simulink model "Multiuav"  (Simulink 4.00)
settings: Solver=FixedStepDiscrete  StartTime=0.0  StopTime=g_StopTime  FixedStep=g_SampleTime  RelTol=1e-3
undefined symbols (not defined in the file): ATRFunctions, g_AssignmentAlgorithm, g_CommandTurnRadius, g_CoordinationDelayDen, g_DefaultWaypointAltitude, g_EnableTarget, g_EnableVehicle, g_EntityTypes, g_MaxNumberTargets, g_MaxNumberVehicles, g_MaxReassignmentDeltaTime, g_ObjectMessageIDs, g_OptionSaveDataAVDS, g_OptionSaveDataPlot, g_SampleTime, g_SensorRollLimitDeg, g_TargetStates, g_Tasks, g_TypeAssignment, g_VehicleInputFiles, g_VehicleMemory, g_VehicleTypes, g_WaypointDefinitions, g_WaypointTypes
libraries: cooperative x42
(part 4 of 4)

== system Multiuav/Vehicles/UAV1/EmbeddedFlightSoftware/CooperationManager/Calculate Assignment/CapTransShip/Assignment for Local Vehicle ==
  note: Assignment for Local Vehicle
      |
      | PURPOSE: Output the target and task assignment
      |      for the local vehicle..
      |
      | IMPLEMENTATION: This block uses a"Selector" Block to select the target and task assignment
      |       based on the VehicleID signal.
  note: Note: new assignment is implemented in the route manager.
  In1 : Inport  Port=1  LatchInput=off  SampleTime=g_SampleTime
  In2 : Inport  Port=2  LatchInput=off  SampleTime=g_SampleTime
  Bus Creator : BusCreator  Inputs=3
  Bus Selector : BusSelector  OutputSignals=VehicleID  MuxedOutput=off
  Constant : Constant  Value=0
  Demux : Demux  Outputs=2  BusSelectionMode=off
  SelectedSignals : MATLABFcn  MATLABFcn=[u(1),g_MaxNumberVehicles+u(1)]  OutputDimensions=-1  OutputSignalType=auto  Output1D=on
  Selector : Selector  InputType=Vector  ElementSrc=External  Elements=[1 3]  RowSrc=Internal  Rows=1  ColumnSrc=Internal  Columns=1  InputPortWidth=2*g_MaxNumberVehicles + 1
  Out1 : Outport  Port=1
  wires:
  In1/1 -> Bus Selector/1
  Bus Creator/1 -> Out1/1  "Assignment - Local"
  Demux/1 -> Bus Creator/1  "Target Assignment - Local"
  Demux/2 -> Bus Creator/2  "Task Assignment  - Local"
  Bus Selector/1 -> SelectedSignals/1  "<VehicleID>"
  In2/1 -> Selector/1
  Constant/1 -> Bus Creator/3  "NewAssignmentFlag"
  SelectedSignals/1 -> Selector/2
  Selector/1 -> Demux/1

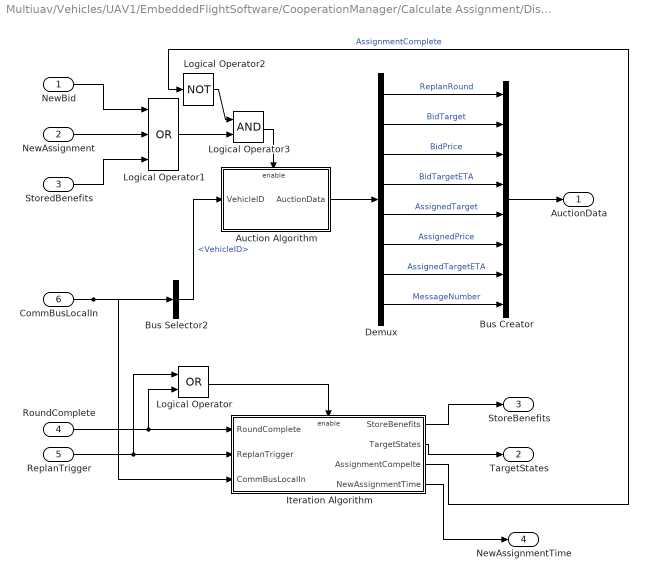
== system Multiuav/Vehicles/UAV1/EmbeddedFlightSoftware/CooperationManager/Calculate Assignment/DistAuctItCapTransShip/Assignment Algorithm ==
  NewBid : Inport  Port=1  LatchInput=off
  NewAssignment : Inport  Port=2  LatchInput=off
  StoredBenefits : Inport  Port=3  LatchInput=off
  RoundComplete : Inport  Port=4  LatchInput=off
  ReplanTrigger : Inport  Port=5  LatchInput=off
  CommBusLocalIn : Inport  Port=6  LatchInput=off
  Auction Algorithm : Subsystem  TreatAsAtomicUnit=on
      settings: RTWFcnNameOpts=Auto  RTWFileNameOpts=Auto
  Bus Creator : BusCreator  Inputs=8
  Bus Selector2 : BusSelector  OutputSignals=VehicleID  MuxedOutput=off
  Demux : Demux  Outputs=[2, g_MaxNumberVehicles,g_MaxNumberVehicles,g_MaxNumberVehicles,g_MaxNumberVehicles,g_MaxNumberVehicles,g_MaxNumberVehicles,1]  BusSelectionMode=off
  Iteration Algorithm : Subsystem  TreatAsAtomicUnit=on
      settings: RTWFcnNameOpts=Auto  RTWFileNameOpts=Auto
  Logical Operator : Logic  Operator=OR  Inputs=2
  Logical Operator1 : Logic  Operator=OR  Inputs=3
  Logical Operator2 : Logic  Operator=NOT  Inputs=21
  Logical Operator3 : Logic  Operator=AND  Inputs=2
  AuctionData : Outport  Port=1
  TargetStates : Outport  Port=2
  StoreBenefits : Outport  Port=3
  NewAssignmentTime : Outport  Port=4
  wires:
  Logical Operator3/1 -> Auction Algorithm/Enable
  Logical Operator2/1 -> Logical Operator3/1
  Logical Operator1/1 -> Logical Operator3/2
  Iteration Algorithm/3(AssignmentCompelte) -> Logical Operator2/1  "AssignmentComplete"
  StoredBenefits/1 -> Logical Operator1/3
  Demux/3 -> Bus Creator/3  "BidPrice"
  Bus Selector2/1 -> Auction Algorithm/1(VehicleID)  "<VehicleID>"
  CommBusLocalIn/1 -> Iteration Algorithm/3(CommBusLocalIn), Bus Selector2/1
  NewBid/1 -> Logical Operator1/1
  NewAssignment/1 -> Logical Operator1/2
  Auction Algorithm/1(AuctionData) -> Demux/1
  Demux/6 -> Bus Creator/6  "AssignedPrice"
  Logical Operator/1 -> Iteration Algorithm/Enable
  RoundComplete/1 -> Logical Operator/2, Iteration Algorithm/1(RoundComplete)
  ReplanTrigger/1 -> Logical Operator/1, Iteration Algorithm/2(ReplanTrigger)
  Iteration Algorithm/2(TargetStates) -> TargetStates/1
  Iteration Algorithm/1(StoreBenefits) -> StoreBenefits/1
  Bus Creator/1 -> AuctionData/1
  Demux/8 -> Bus Creator/8  "MessageNumber"
  Demux/5 -> Bus Creator/5  "AssignedTarget"
  Demux/4 -> Bus Creator/4  "BidTargetETA"
  Demux/2 -> Bus Creator/2  "BidTarget"
  Demux/1 -> Bus Creator/1  "ReplanRound"
  Demux/7 -> Bus Creator/7  "AssignedTargetETA"
  Iteration Algorithm/4(NewAssignmentTime) -> NewAssignmentTime/1

== system Multiuav/Vehicles/UAV1/EmbeddedFlightSoftware/CooperationManager/Calculate Assignment/DistAuctItCapTransShip/Message Processing ==
  CommBusIn : Inport  Port=1  LatchInput=off
  SimBusIn : Inport  Port=2  LatchInput=off
  CommBusLocalIn : Inport  Port=3  LatchInput=off
  ReplanTrigger : Inport  Port=4  LatchInput=off
  Bus Selector1 : BusSelector  OutputSignals=AuctionData  MuxedOutput=off
  Bus Selector2 : BusSelector  OutputSignals=VehicleID  MuxedOutput=off
  Bus Selector4 : BusSelector  OutputSignals=ExternalTruth.VehicleIsDead  MuxedOutput=on
  Demux : Demux  Outputs=[1 1 1]  BusSelectionMode=off
  Logical Operator : Logic  Operator=NOT  Inputs=2
  Mux1 : Mux  Inputs=4
  S-Function : S-Function  FunctionName=DAINF_MessageControlS  PortCounts=[]  SFunctionModules=''
  NewBid : Outport  Port=1
  NewAssignment : Outport  Port=2
  RoundComplete : Outport  Port=3
  wires:
  Demux/3 -> RoundComplete/1
  Demux/2 -> NewAssignment/1
  Demux/1 -> NewBid/1
  S-Function/1 -> Demux/1
  Mux1/1 -> S-Function/1
  Bus Selector2/1 -> Mux1/1  "<VehicleID>"
  CommBusLocalIn/1 -> Bus Selector2/1
  Logical Operator/1 -> Mux1/2  "ActiveVehicles"
  ReplanTrigger/1 -> Mux1/4  "ReplanTrigger"
  Bus Selector1/1 -> Mux1/3  "<AuctionData>"
  CommBusIn/1 -> Bus Selector1/1
  Bus Selector4/1 -> Logical Operator/1  "<VehicleIsDead>"
  SimBusIn/1 -> Bus Selector4/1

== system Multiuav/Vehicles/UAV1/EmbeddedFlightSoftware/CooperationManager/Calculate Assignment/DistAuctItCapTransShip/Replan Logic ==
  EnableType : Inport  Port=1  LatchInput=off
  Constant : Constant  Value=1
  Constant1 : Constant  Value=1
  Constant2 : Constant  Value=0
  Multiport Switch : MultiPortSwitch  Inputs=4
  Sum : Sum  Inputs=++|  SaturateOnIntegerOverflow=on
  ReplanTrigger : Outport  Port=1
  wires:
  Constant1/1 -> Multiport Switch/5, Multiport Switch/3
  Constant2/1 -> Multiport Switch/4, Multiport Switch/2
  Multiport Switch/1 -> ReplanTrigger/1
  Sum/1 -> Multiport Switch/1
  Constant/1 -> Sum/1
  EnableType/1 -> Sum/2

== system Multiuav/Vehicles/UAV1/EmbeddedFlightSoftware/CooperationManager/Calculate Assignment/DistAuctItCapTransShip/Store Benefits ==
  CommBusIn : Inport  Port=1  LatchInput=off
  CommBusLocalIn : Inport  Port=2  LatchInput=off
  TargetStates : Inport  Port=3  LatchInput=off
  Enable : EnablePort  ShowOutputPort=on
  Demux : Demux  Outputs=[g_MaxNumberTargets,g_MaxNumberTargets,1]  BusSelectionMode=off
  Mux : Mux  Inputs=5
  Mux1 : Mux  Inputs=10
  S-Function : S-Function  FunctionName=DINF_CalculateBenefitsS  Parameters=g_MaxNumberTargets,g_MaxNumberVehicles  PortCounts=[]  SFunctionModules=''
  S-Function1 : S-Function  Orientation=left  FunctionName=DAINF_StoreBenefitsS  PortCounts=[]  SFunctionModules=''
  SimBusSelector : BusSelector  OutputSignals=Time,VehicleID,Dynamics(com).AC Dynamics.Position_x,Dynamics(com).AC Dynamics.Position_y,Dynamics(com).AC Dynamics.Psi,Dynamics(com).TacticalManuevering.WayPointNumber,EFS(com).TargetManager(com).SensedTargetInformation.Targets,EFS(com).SensorManager(com).ATR Combined.Desired Headings  MuxedOutput=off
  SimBusSelector1 : BusSelector  OutputSignals=VehicleID  MuxedOutput=off
  SimBusSelector2 : BusSelector  OutputSignals=TriggerReplan  MuxedOutput=off
  BenefitsStored : Outport  Port=1  OutputWhenDisabled=reset  InitialOutput=[0]
  wires:
  SimBusSelector2/1 -> Mux1/10  "<TriggerReplan>"
  CommBusIn/1 -> SimBusSelector2/1
  Enable/1 -> BenefitsStored/1
  SimBusSelector1/1 -> Mux/1  "<VehicleID>"
  Mux/1 -> S-Function1/1
  TargetStates/1 -> Mux/5, Mux1/9  "TargetStates"
  SimBusSelector/6 -> Mux1/6  "<WayPointNumber>"
  SimBusSelector/8 -> Mux1/8  "<Desired Headings>"
  SimBusSelector/7 -> Mux1/7  "<Targets>"
  SimBusSelector/5 -> Mux1/5  "<Psi>"
  SimBusSelector/4 -> Mux1/4  "<Position_y>"
  SimBusSelector/3 -> Mux1/3  "<Position_x>"
  SimBusSelector/2 -> Mux1/2  "<VehicleID>"
  SimBusSelector/1 -> Mux1/1  "<Time>"
  CommBusLocalIn/1 -> SimBusSelector1/1, SimBusSelector/1
  Mux1/1 -> S-Function/1
  S-Function/1 -> Demux/1
  Demux/3 -> Mux/4  "SearchBenefit"
  Demux/2 -> Mux/3  "TimeToComplete"
  Demux/1 -> Mux/2  "TaskBenefits"

== system Multiuav/Vehicles/UAV1/EmbeddedFlightSoftware/CooperationManager/Calculate Assignment/DistItCapTransShip/Assignment Algorithm ==
  ActiveVehicles : Inport  Port=1  LatchInput=off
  ReplanRoundIn : Inport  Port=2  LatchInput=off
  TargetStatesIn : Inport  Port=3  LatchInput=off
  TaskBenefits : Inport  Port=4  LatchInput=off
  TimeToComplete : Inport  Port=5  LatchInput=off
  SearchBenefits : Inport  Port=6  LatchInput=off
  Sync : Inport  Port=7  LatchInput=off
  ReplanTrigger : Inport  Port=8  LatchInput=off
  CommBusLocalIn : Inport  Port=9  LatchInput=off
  Bus Selector : BusSelector  OutputSignals=VehicleID,EFS(com).TargetManager(com).Target Status.TargetStatus,Dynamics(com).TacticalManuevering.WayPointNumber,Dynamics(com).AC Dynamics.Position_x,Dynamics(com).AC Dynamics.Position_y,Dynamics(com).AC Dynamics.Psi  MuxedOutput=off
  Demux : Demux  Outputs=[2 g_MaxNumberTargets 1 1]  BusSelectionMode=off
  Mux : Mux  Inputs=14
  S-Function : S-Function  FunctionName=DINF_CapTransShipAssignS  Parameters=g_MaxNumberTargets,g_MaxNumberVehicles  PortCounts=[]  SFunctionModules=''
  TargetStatesOut : Outport  Port=1
  ReplanRoundOut : Outport  Port=2
  SendBenefitsTrigger : Outport  Port=3
  NewAssignmentTime : Outport  Port=4
  wires:
  Demux/3 -> SendBenefitsTrigger/1
  Bus Selector/6 -> Mux/14  "<Psi>"
  Bus Selector/5 -> Mux/13  "<Position_y>"
  Bus Selector/4 -> Mux/12  "<Position_x>"
  Bus Selector/3 -> Mux/11  "<WayPointNumber>"
  Bus Selector/2 -> Mux/10  "<TargetStatus>"
  Bus Selector/1 -> Mux/9  "<VehicleID>"
  CommBusLocalIn/1 -> Bus Selector/1
  Demux/1 -> ReplanRoundOut/1
  Demux/2 -> TargetStatesOut/1
  S-Function/1 -> Demux/1
  Mux/1 -> S-Function/1
  ReplanTrigger/1 -> Mux/8
  Sync/1 -> Mux/7
  SearchBenefits/1 -> Mux/6
  TimeToComplete/1 -> Mux/5
  TaskBenefits/1 -> Mux/4
  TargetStatesIn/1 -> Mux/3
  ReplanRoundIn/1 -> Mux/2
  ActiveVehicles/1 -> Mux/1
  Demux/4 -> NewAssignmentTime/1

== system Multiuav/Vehicles/UAV1/EmbeddedFlightSoftware/CooperationManager/Calculate Assignment/DistItCapTransShip/Iteration Logic ==
  CommBusIn : Inport  Port=1  LatchInput=off
  SimBusIn : Inport  Port=2  LatchInput=off
  Bus Selector : BusSelector  OutputSignals=ExternalTruth.VehicleIsDead  MuxedOutput=on
  Bus Selector1 : BusSelector  OutputSignals=TaskBenefits  MuxedOutput=off
  Demux : Demux  Outputs=[2,g_MaxNumberTargets,g_MaxNumberVehicles*g_MaxNumberTargets,g_MaxNumberVehicles*g_MaxNumberTargets,g_MaxNumberVehicles,1]  BusSelectionMode=off
  Logical Operator : Logic  Operator=NOT  Inputs=2
  Mux1 : Mux  Inputs=2
  S-Function : S-Function  FunctionName=DINF_ComparePlanS  Parameters=g_MaxNumberVehicles,g_MaxNumberTargets  PortCounts=[]  SFunctionModules=''
  ActiveVehicles : Outport  Port=1
  ReplanRound : Outport  Port=2
  TargetStates : Outport  Port=3
  TaskBenefits : Outport  Port=4
  TimeToComplete : Outport  Port=5
  SearchBenefits : Outport  Port=6
  Sync : Outport  Port=7
  wires:
  Demux/6 -> Sync/1
  Demux/5 -> SearchBenefits/1
  Demux/4 -> TimeToComplete/1
  Demux/3 -> TaskBenefits/1
  Demux/2 -> TargetStates/1
  Demux/1 -> ReplanRound/1
  S-Function/1 -> Demux/1
  Mux1/1 -> S-Function/1
  Bus Selector1/1 -> Mux1/2  "<TaskBenefits>"
  CommBusIn/1 -> Bus Selector1/1
  Logical Operator/1 -> ActiveVehicles/1, Mux1/1
  SimBusIn/1 -> Bus Selector/1
  Bus Selector/1 -> Logical Operator/1  "<VehicleIsDead>"

== system Multiuav/Vehicles/UAV1/EmbeddedFlightSoftware/CooperationManager/Calculate Assignment/DistItCapTransShip/Replan Logic ==
  EnableType : Inport  Port=1  LatchInput=off
  Constant : Constant  Value=1
  Constant1 : Constant  Value=1
  Constant2 : Constant  Value=0
  Multiport Switch : MultiPortSwitch  Inputs=4
  Sum : Sum  Inputs=++|  SaturateOnIntegerOverflow=on
  ReplanTrigger : Outport  Port=1
  wires:
  Constant1/1 -> Multiport Switch/5, Multiport Switch/3
  Constant2/1 -> Multiport Switch/4, Multiport Switch/2
  Multiport Switch/1 -> ReplanTrigger/1
  Sum/1 -> Multiport Switch/1
  Constant/1 -> Sum/1
  EnableType/1 -> Sum/2

== system Multiuav/Vehicles/UAV1/EmbeddedFlightSoftware/CooperationManager/Calculate Assignment/DistItCapTransShip/Send Benefits ==
  CommBusIn : Inport  Port=1  LatchInput=off
  CommBusLocalIn : Inport  Port=2  LatchInput=off
  TargetStates : Inport  Port=3  LatchInput=off
  ReplanRound : Inport  Port=4  LatchInput=off
  Enable : EnablePort
  Bus Creator : BusCreator  Inputs=5
  Demux : Demux  Outputs=[g_MaxNumberTargets,g_MaxNumberTargets,1]  BusSelectionMode=off
  Mux1 : Mux  Inputs=10
  S-Function : S-Function  FunctionName=DINF_CalculateBenefitsS  Parameters=g_MaxNumberTargets,g_MaxNumberVehicles  PortCounts=[]  SFunctionModules=''
  SimBusSelector : BusSelector  OutputSignals=Time,VehicleID,Dynamics(com).AC Dynamics.Position_x,Dynamics(com).AC Dynamics.Position_y,Dynamics(com).AC Dynamics.Psi,Dynamics(com).TacticalManuevering.WayPointNumber,EFS(com).TargetManager(com).SensedTargetInformation.Targets,EFS(com).SensorManager(com).ATR Combined.Desired Headings  MuxedOutput=off
  SimBusSelector1 : BusSelector  OutputSignals=TriggerReplan  MuxedOutput=off
  Algorithm Data : Outport  Port=1
  wires:
  SimBusSelector1/1 -> Mux1/10  "<TriggerReplan>"
  CommBusIn/1 -> SimBusSelector1/1
  SimBusSelector/6 -> Mux1/6  "<WayPointNumber>"
  ReplanRound/1 -> Bus Creator/1  "ReplanRound"
  TargetStates/1 -> Mux1/9, Bus Creator/2  "TargetStates"
  SimBusSelector/8 -> Mux1/8  "<Desired Headings>"
  SimBusSelector/7 -> Mux1/7  "<Targets>"
  SimBusSelector/5 -> Mux1/5  "<Psi>"
  SimBusSelector/4 -> Mux1/4  "<Position_y>"
  SimBusSelector/3 -> Mux1/3  "<Position_x>"
  SimBusSelector/2 -> Mux1/2  "<VehicleID>"
  SimBusSelector/1 -> Mux1/1  "<Time>"
  CommBusLocalIn/1 -> SimBusSelector/1
  Mux1/1 -> S-Function/1
  S-Function/1 -> Demux/1
  Demux/3 -> Bus Creator/5  "SearchBenefit"
  Demux/2 -> Bus Creator/4  "TimeToComplete"
  Bus Creator/1 -> Algorithm Data/1  "Algorithm Data"
  Demux/1 -> Bus Creator/3  "TaskBenefits"

== system Multiuav/Vehicles/UAV1/EmbeddedFlightSoftware/RouteManager/Task Status/D Latch/D Latch ==
  D : Inport  Port=1  LatchInput=off
  C : EnablePort
  Q : Outport  Port=1  InitialOutput=g_Tasks.Undefined
  wires:
  D/1 -> Q/1

== system Multiuav/Vehicles/UAV1/EmbeddedFlightSoftware/RouteManager/Task Status/D Latch1/D Latch ==
  D : Inport  Port=1  LatchInput=off
  C : EnablePort
  Q : Outport  Port=1  InitialOutput=0
  wires:
  D/1 -> Q/1

== system Multiuav/Vehicles/UAV1/EmbeddedFlightSoftware/RouteManager/Task Status/D Latch2/D Latch ==
  D : Inport  Port=1  LatchInput=off
  C : EnablePort
  Q : Outport  Port=1  InitialOutput=0
  wires:
  D/1 -> Q/1

== system Multiuav/Vehicles/UAV1/EmbeddedFlightSoftware/RouteManager/Task Status/Task Failed Check/Task Failed Check ==
  Local (Comm) : Inport  Port=1  LatchInput=off
  LastTargetState : Inport  Port=2  LatchInput=off
  Enable : EnablePort
  Bus Selector6 : BusSelector  OutputSignals=VehicleID,Dynamics(com).TacticalManuevering.AssignedTarget,Dynamics(com).TacticalManuevering.WayPointTypeCurrent,EFS(com).TargetManager(com).Target Status.TargetStatus,Dynamics(com).TacticalManuevering.WayPointNumber  MuxedOutput=off
  Mux1 : Mux  Inputs=7
  Save Last Task : DataStoreWrite  DataStoreName=LastWaypointType  SampleTime=g_SampleTime
  SaveLastTargetState : DataStoreWrite  DataStoreName=LastTargetState  SampleTime=g_SampleTime
  TargetStatusS : S-Function  FunctionName=TaskFailedS  Parameters=g_MaxNumberTargets  PortCounts=[]  SFunctionModules=''
  Unit Delay : UnitDelay  X0=0  SampleTime=g_SampleTime
      settings: RTWStateStorageClass=Auto
  Unit Delay1 : UnitDelay  X0=0  SampleTime=g_SampleTime
      settings: RTWStateStorageClass=Auto
  TaskFailed : Outport  Port=1
  wires:
  Bus Selector6/5 -> Mux1/7  "<WayPointNumber>"
  LastTargetState/1 -> Mux1/6
  Bus Selector6/4 -> Mux1/5, SaveLastTargetState/1  "<TargetStatus>"
  Unit Delay1/1 -> Mux1/3
  Bus Selector6/1 -> Mux1/1  "<VehicleID>"
  Unit Delay/1 -> Mux1/2
  TargetStatusS/1 -> TaskFailed/1
  Mux1/1 -> TargetStatusS/1
  Bus Selector6/2 -> Unit Delay/1  "<AssignedTarget>"
  Local (Comm)/1 -> Bus Selector6/1
  Bus Selector6/3 -> Mux1/4, Unit Delay1/1, Save Last Task/1  "<WayPointTypeCurrent>"

== system Multiuav/Vehicles/UAV1/EmbeddedFlightSoftware/SensorManager/ATR Single/SingleATR/Assume Responsibility ==
  NewTargets : Inport  Port=1  LatchInput=off
  VehicleID : Inport  Port=2  LatchInput=off
  Enable : EnablePort
  Mux : Mux  Inputs=2
  S-Function : S-Function  FunctionName=DAINF_AssumeDutyS  PortCounts=[]  SFunctionModules=''
  wires:
  NewTargets/1 -> Mux/2
  VehicleID/1 -> Mux/1
  Mux/1 -> S-Function/1

== system Multiuav/Vehicles/UAV1/EmbeddedFlightSoftware/CooperationManager/Calculate Assignment/DistAuctItCapTransShip/Assignment Algorithm/Auction Algorithm ==
  VehicleID : Inport  Port=1  LatchInput=off
  Enable : EnablePort  StatesWhenEnabling=reset
  Auction Algorithm : S-Function  FunctionName=DAINF_AuctionS  PortCounts=[]  SFunctionModules=''
  AuctionData : Outport  Port=1
  wires:
  VehicleID/1 -> Auction Algorithm/1
  Auction Algorithm/1 -> AuctionData/1

== system Multiuav/Vehicles/UAV1/EmbeddedFlightSoftware/CooperationManager/Calculate Assignment/DistAuctItCapTransShip/Assignment Algorithm/Iteration Algorithm ==
  RoundComplete : Inport  Port=1  LatchInput=off
  ReplanTrigger : Inport  Port=2  LatchInput=off
  CommBusLocalIn : Inport  Port=3  LatchInput=off
  Enable : EnablePort  StatesWhenEnabling=reset
  Bus Selector : BusSelector  OutputSignals=VehicleID,EFS(com).TargetManager(com).Target Status.TargetStatus,Dynamics(com).TacticalManuevering.WayPointNumber,Dynamics(com).AC Dynamics.Position_x,Dynamics(com).AC Dynamics.Position_y,Dynamics(com).AC Dynamics.Psi  MuxedOutput=off
  Demux : Demux  Outputs=[g_MaxNumberTargets,1,1,1]  BusSelectionMode=off
  Iteration Algorithm : S-Function  FunctionName=DAINF_IterationControlS  PortCounts=[]  SFunctionModules=''
  Mux : Mux  Inputs=8
  StoreBenefits : Outport  Port=1  OutputWhenDisabled=reset  InitialOutput=[0]
  TargetStates : Outport  Port=2
  AssignmentCompelte : Outport  Port=3  OutputWhenDisabled=reset  InitialOutput=[0]
  NewAssignmentTime : Outport  Port=4  OutputWhenDisabled=reset  InitialOutput=[0]
  wires:
  Demux/3 -> AssignmentCompelte/1
  Bus Selector/6 -> Mux/8  "<Psi>"
  Bus Selector/5 -> Mux/7  "<Position_y>"
  Bus Selector/4 -> Mux/6  "<Position_x>"
  Bus Selector/3 -> Mux/5  "<WayPointNumber>"
  Bus Selector/2 -> Mux/4  "<TargetStatus>"
  Bus Selector/1 -> Mux/3  "<VehicleID>"
  Demux/2 -> StoreBenefits/1
  CommBusLocalIn/1 -> Bus Selector/1
  Mux/1 -> Iteration Algorithm/1
  ReplanTrigger/1 -> Mux/2
  RoundComplete/1 -> Mux/1
  Demux/1 -> TargetStates/1
  Iteration Algorithm/1 -> Demux/1
  Demux/4 -> NewAssignmentTime/1
